simulink model "huamo"  (R2014a)
settings: Solver=ode3  SolverMode=SingleTasking  StartTime=0.0  StopTime=10.0  RelTol=1e-3
PreLoadFcn:
  | waijung.modelPreload; % Required for working with Waijung Blockset. Do not remove.
undefined symbols (not defined in the file): ARM, dfilt, DiscIntNeverNeededParam, fdesignblkfcn, gcbh, Link, LQFP64, MDK, ST, STM32F405RG
libraries: simulink x33, stm32f4_io_lib x3, stm32f4_device_config_lib x2, dsparch4 x2
(part 2 of 6)

== system huamo/IMU ==
  Bus Creator : BusCreator  Inputs=3
  Cal : Subsystem  TreatAsAtomicUnit=on
  Gain{1..4} (4 alike) : Gain  Gain=-1
  Mux : Mux  Inputs=3
  Mux1 : Mux  Inputs=3
  angle : S-Function  Priority=1  FunctionName=stm32f4_usart  Parameters=configuration,uartmodule,transfer,baudrate,inputtype,outputtype,confstr,binheaderarray,binterminatorarray,asciiheader,asciiterminator,bindatalength,packetmode,varname,sampletime,sampletimestr,blockid  EnableBusSupport=off  mask(stm32f4_usart){configuration=Rx, uartmodule=3, baudrate=115200, databits=8, parity=No, stopbit=1, remaptxpin=Not used, remaprxpin=Not used, flowcontrol=None, remapctspin=Not used, remaprtspin=Not used, advanceoptions=off, rxbuffersize=512, txbuffersize=512, transfer=Non-Blocking, packetmode=Binary, binheader='A5 5A 11 A4', binterminator='AA', porttype_double=0, porttype_single=0, porttype_int8=0, porttype_uint8=14, porttype_int16=0, porttype_uint16=0, porttype_int32=0, porttype_uint32=0, asciiformat='value=%d,%f', rx_asciiterminator=CRLF (0x0D 0x0A - "\r\n"), tx_asciiterminator=LF (0x0A - "\n"), storagename=<empty>, varname=, inputtype=[0], outputtype=[15 3  3 3 3 3 3 3 3 3 3 3 3 3 3 3], binheaderarray=[4 165   90   17  164    0    0    0    0    0    0    0    0    0    0    0    0    0    0    0    0    0    0    0    0], binterminatorarray=[1 170], bindatalength=14, asciiheader='value=%d,%f\r\n', asciiterminator=[2 13 10], sampletime=-1, sampletimestr=0.005, blockid=IMUangle, confstr=[ "dummy", "0", "*", "*", "0", "*", "*", "0", "*", "*", "0", "*", "*", "1", "4", "3", "1", "4", "1", "512", "512", "1", "3", "115200", "8", "No", "1", "None", "USART3"], lastmodule=1}
      mask prompts: uartmodule "UART Module"; baudrate "Baud rate (bps)"; databits "Data bits"; stopbit "Stop bit"; remaptxpin "Tx Pin"; remaprxpin "Rx Pin"; flowcontrol "Hardware flow control"; remapctspin "HW Flow control, CTS Pin"; remaprtspin "HW Flow control, RTS Pin"; advanceoptions "Advance options"; rxbuffersize "Rx buffer size (bytes)"; txbuffersize "Tx buffer size (bytes)"; packetmode "Packet mode"; binheader "Binary header (example: '7E 7E')"; binterminator "Binary terminator (example: '03 03')"; porttype_double "Number of data port, type DOUBLE"; porttype_single "Number of data port, type SINGLE"; porttype_int8 "Number of data port, type INT8"; porttype_uint8 "Number of data port, type UINT8"; porttype_int16 "Number of data port, type INT16"; porttype_uint16 "Number of data port, type UINT16"; porttype_int32 "Number of data port, type INT32"; porttype_uint32 "Number of data port, type UINT32"; asciiformat "Ascii format"; rx_asciiterminator "End of packet"; tx_asciiterminator "End of packet"; storagename "Buffer"; varname "Var name"; inputtype "Input data type"; outputtype "Output data type"; binheaderarray "Binary header"; binterminatorarray "Binary terminator"; bindatalength "Binary data length"; asciiheader "Ascii header (printf format)"; asciiterminator "Ascii terminator"; sampletime "Sample time (sec)"; sampletimestr "Compiled sample time (sec) in string"; confstr "Configuration string"; lastmodule "Last module selected"
      mask help:
      | Data type for Ascii format
      | %u, %i, %d, %o, %x: uint32
      | %e, %g, %f: single
      | %c: int8
      mask init:
      | stm32f4_usart_callback('init');
      mask Help: web(fullfile(waijungdocroot,'stm32f4_usart_rx.htm'), '-browser')
      mask TypeOptions configuration: Setup | Tx | Rx
      mask Callback configuration: stm32f4_usart_callback('configuration');
      mask TypeOptions uartmodule: 1 | 2 | 3 | 4 | 5 | 6
      mask Callback uartmodule: stm32f4_usart_callback('uartmodule');
      mask Callback baudrate: stm32f4_usart_callback('baudrate');
      mask TypeOptions databits: 8
      mask TypeOptions parity: No | Odd | Even
      mask TypeOptions stopbit: 0.5 | 1 | 1.5 | 2
      mask TypeOptions remaptxpin: Not used | A9 | B6
      mask TypeOptions remaprxpin: Not used | A10 | B7
      mask TypeOptions flowcontrol: None | RTS | CTS | RTS/CTS
      mask Callback flowcontrol: stm32f4_usart_callback('flowcontrol');
      mask TypeOptions remapctspin: Not used | A11
      mask TypeOptions remaprtspin: Not used | A12
      mask Callback advanceoptions: stm32f4_usart_callback('advanceoptions');
      mask TypeOptions rxbuffersize: 16 | 32 | 64 | 128 | 256 | 512 | 1024 | 2048
      mask TypeOptions txbuffersize: 16 | 32 | 64 | 128 | 256 | 512 | 1024 | 2048
      mask TypeOptions transfer: Blocking | Non-Blocking
      mask Callback transfer: stm32f4_usart_callback('transfer');
      mask TypeOptions packetmode: Ascii | Binary | String Buffer
      mask Callback packetmode: stm32f4_usart_callback('packetmode');
      mask Callback binheader: stm32f4_usart_callback('binheader');
      mask Callback binterminator: stm32f4_usart_callback('binterminator');
      mask Callback porttype_double: stm32f4_usart_callback('porttype');
      mask Callback porttype_single: stm32f4_usart_callback('porttype');
      mask Callback porttype_int8: stm32f4_usart_callback('porttype');
      mask Callback porttype_uint8: stm32f4_usart_callback('porttype');
      mask Callback porttype_int16: stm32f4_usart_callback('porttype');
      mask Callback porttype_uint16: stm32f4_usart_callback('porttype');
      mask Callback porttype_int32: stm32f4_usart_callback('porttype');
      mask Callback porttype_uint32: stm32f4_usart_callback('porttype');
      mask Callback asciiformat: stm32f4_usart_callback('asciiformat');
      mask TypeOptions rx_asciiterminator: CR (0x0D - "\r") | LF (0x0A - "\n") | CRLF (0x0D 0x0A - "\r\n")
      mask Callback rx_asciiterminator: stm32f4_usart_callback('rx_asciiterminator');
      mask TypeOptions tx_asciiterminator: CR (0x0D - "\r") | LF (0x0A - "\n") | CRLF (0x0D 0x0A - "\r\n") | None
      mask Callback tx_asciiterminator: stm32f4_usart_callback('tx_asciiterminator');
      mask TypeOptions storagename: <empty>
      mask Callback storagename: stm32f4_usart_callback('storagename');
      mask Callback varname: stm32f4_usart_callback('varname');
      mask Callback sampletime: stm32f4_usart_callback('sampletime');
      mask Callback sampletimestr: stm32f4_usart_callback('sampletimestr');
      mask Callback blockid: stm32f4_usart_callback('blockid');
      mask Display: text(0.05, 0.5, 'Module: USART3_Rx\nPacket: Binary\nTransfer: Non-Blocking\nTs (sec): 0.005','ver','middle','hor','left'); port_label('output', 1,'READY'); port_label('output', 2,'uint8'); port_label('output', 3,'uint8'); port_label('output', 4,'uint8'); port_label('output', 5,'uint8'); port_label('output', 6,'uint8'); port_label('output', 7,'uint8'); port_label('output', 8,'uint8'); port_label('output', 9,'uint8'); port_label('output', 10,'uint8'); port_label('output', 11,'uint8'); port_label('output', 12,'uint8'); port_label('output', 13,'uint8'); port_label('output', 14,'uint8'); port_label('output', 15,'uint8');
  ANGLE ENABLE : Outport
  IMU BUS : Outport  Port=2
  IMU : Outport  Port=3
  wires:
  angle/1 -> ANGLE ENABLE/1, Cal/Enable
  [alt] -> Bus Creator/3  "alt"
  [Angle_rate] -> Bus Creator/2  "Angle_rate"
  Mux/1 -> [Angle]  "angle"
  [Angle] -> Bus Creator/1  "Angle"
  Cal/2(pitch) -> Gain1/1
  Bus Creator/1 -> IMU BUS/1
  Gain2/1 -> Mux/3
  angle/2 -> Cal/1(yaw_H)
  angle/3 -> Cal/2(yaw_L)
  angle/4 -> Cal/3(pitch_H)
  angle/5 -> Cal/4(pitch_L)
  angle/6 -> Cal/5(roll_H)
  angle/7 -> Cal/6(roll_L)
  angle/8 -> Cal/7(p_H)
  angle/9 -> Cal/8(p_L)
  angle/10 -> Cal/9(q_H)
  angle/11 -> Cal/10(q_L)
  angle/12 -> Cal/11(r_H)
  angle/13 -> Cal/12(r_L)
  angle/14 -> Cal/13(alt_H)
  angle/15 -> Cal/14(alt_L)
  Gain1/1 -> Mux/2
  Mux1/1 -> [Angle_rate]  "angle"
  Cal/6(r) -> Gain4/1
  Cal/5(q) -> Gain3/1
  Cal/4(p) -> Mux1/1
  Gain4/1 -> Mux1/3
  Gain3/1 -> Mux1/2
  Cal/3(roll) -> Mux/1
  Cal/1(yaw) -> Gain2/1
  Cal/7(alt) -> [alt]
  Cal/8(out) -> IMU/1

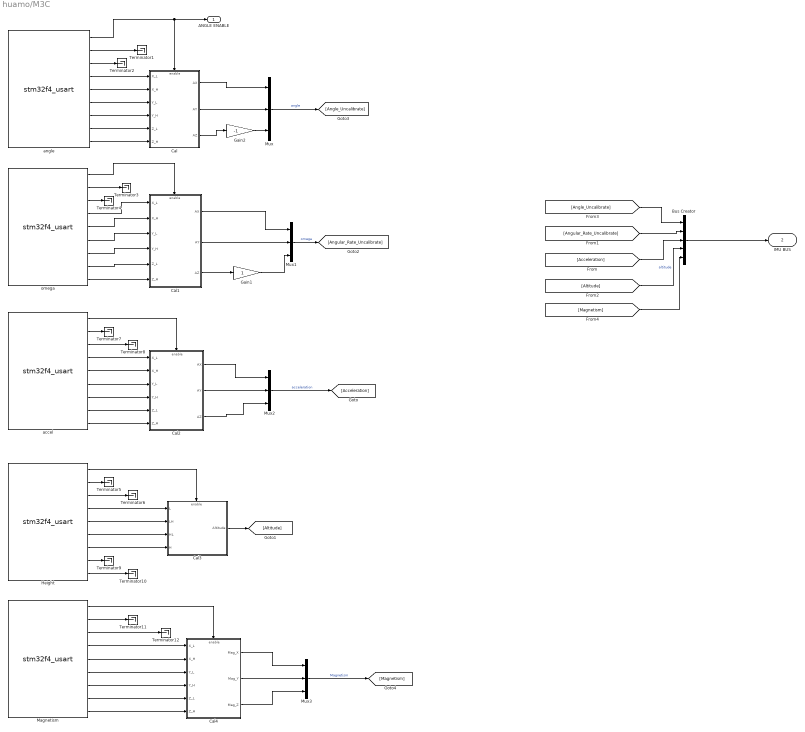
== system huamo/M3C ==
  Bus Creator : BusCreator  Inputs=5
  Cal : Subsystem  TreatAsAtomicUnit=on
  Cal1 : Subsystem  TreatAsAtomicUnit=on
  Cal2 : Subsystem  TreatAsAtomicUnit=on
  Cal3 : Subsystem  TreatAsAtomicUnit=on
  Cal4 : Subsystem  TreatAsAtomicUnit=on
  Gain1 : Gain
  Gain2 : Gain  Gain=-1
  Height : S-Function  Priority=1  FunctionName=stm32f4_usart  Parameters=configuration,uartmodule,transfer,baudrate,inputtype,outputtype,confstr,binheaderarray,binterminatorarray,asciiheader,asciiterminator,bindatalength,packetmode,varname,sampletime,sampletimestr,blockid  EnableBusSupport=off  mask(stm32f4_usart){configuration=Rx, uartmodule=3, baudrate=115200, databits=8, parity=No, stopbit=1, remaptxpin=Not used, remaprxpin=Not used, flowcontrol=None, remapctspin=Not used, remaprtspin=Not used, advanceoptions=off, rxbuffersize=512, txbuffersize=512, transfer=Non-Blocking, packetmode=Binary, binheader='A7 7A 75', binterminator='', porttype_double=0, porttype_single=0, porttype_int8=0, porttype_uint8=8, porttype_int16=0, porttype_uint16=0, porttype_int32=0, porttype_uint32=0, asciiformat='value=%d,%f', rx_asciiterminator=CRLF (0x0D 0x0A - "\r\n"), tx_asciiterminator=LF (0x0A - "\n"), storagename=<empty>, varname=, inputtype=[0], outputtype=[9 3  3 3 3 3 3 3 3 3], binheaderarray=[3 167  122  117    0    0    0], binterminatorarray=[0 ], bindatalength=8, asciiheader='value=%d,%f\r\n', asciiterminator=[2 13 10], sampletime=-1, sampletimestr=0.005, blockid=M3CHeight, confstr=[ "dummy", "0", "*", "*", "0", "*", "*", "0", "*", "*", "0", "*", "*", "1", "4", "3", "1", "4", "1", "512", "512", "1", "3", "115200", "8", "No", "1", "None", "USART3"], lastmodule=1}
      mask prompts: uartmodule "UART Module"; baudrate "Baud rate (bps)"; databits "Data bits"; stopbit "Stop bit"; remaptxpin "Tx Pin"; remaprxpin "Rx Pin"; flowcontrol "Hardware flow control"; remapctspin "HW Flow control, CTS Pin"; remaprtspin "HW Flow control, RTS Pin"; advanceoptions "Advance options"; rxbuffersize "Rx buffer size (bytes)"; txbuffersize "Tx buffer size (bytes)"; packetmode "Packet mode"; binheader "Binary header (example: '7E 7E')"; binterminator "Binary terminator (example: '03 03')"; porttype_double "Number of data port, type DOUBLE"; porttype_single "Number of data port, type SINGLE"; porttype_int8 "Number of data port, type INT8"; porttype_uint8 "Number of data port, type UINT8"; porttype_int16 "Number of data port, type INT16"; porttype_uint16 "Number of data port, type UINT16"; porttype_int32 "Number of data port, type INT32"; porttype_uint32 "Number of data port, type UINT32"; asciiformat "Ascii format"; rx_asciiterminator "End of packet"; tx_asciiterminator "End of packet"; storagename "Buffer"; varname "Var name"; inputtype "Input data type"; outputtype "Output data type"; binheaderarray "Binary header"; binterminatorarray "Binary terminator"; bindatalength "Binary data length"; asciiheader "Ascii header (printf format)"; asciiterminator "Ascii terminator"; sampletime "Sample time (sec)"; sampletimestr "Compiled sample time (sec) in string"; confstr "Configuration string"; lastmodule "Last module selected"
      mask help:
      | Data type for Ascii format
      | %u, %i, %d, %o, %x: uint32
      | %e, %g, %f: single
      | %c: int8
      mask init:
      | stm32f4_usart_callback('init');
      mask Help: web(fullfile(waijungdocroot,'stm32f4_usart_rx.htm'), '-browser')
      mask TypeOptions configuration: Setup | Tx | Rx
      mask Callback configuration: stm32f4_usart_callback('configuration');
      mask TypeOptions uartmodule: 1 | 2 | 3 | 4 | 5 | 6
      mask Callback uartmodule: stm32f4_usart_callback('uartmodule');
      mask Callback baudrate: stm32f4_usart_callback('baudrate');
      mask TypeOptions databits: 8
      mask TypeOptions parity: No | Odd | Even
      mask TypeOptions stopbit: 0.5 | 1 | 1.5 | 2
      mask TypeOptions remaptxpin: Not used | A9 | B6
      mask TypeOptions remaprxpin: Not used | A10 | B7
      mask TypeOptions flowcontrol: None | RTS | CTS | RTS/CTS
      mask Callback flowcontrol: stm32f4_usart_callback('flowcontrol');
      mask TypeOptions remapctspin: Not used | A11
      mask TypeOptions remaprtspin: Not used | A12
      mask Callback advanceoptions: stm32f4_usart_callback('advanceoptions');
      mask TypeOptions rxbuffersize: 16 | 32 | 64 | 128 | 256 | 512 | 1024 | 2048
      mask TypeOptions txbuffersize: 16 | 32 | 64 | 128 | 256 | 512 | 1024 | 2048
      mask TypeOptions transfer: Blocking | Non-Blocking
      mask Callback transfer: stm32f4_usart_callback('transfer');
      mask TypeOptions packetmode: Ascii | Binary | String Buffer
      mask Callback packetmode: stm32f4_usart_callback('packetmode');
      mask Callback binheader: stm32f4_usart_callback('binheader');
      mask Callback binterminator: stm32f4_usart_callback('binterminator');
      mask Callback porttype_double: stm32f4_usart_callback('porttype');
      mask Callback porttype_single: stm32f4_usart_callback('porttype');
      mask Callback porttype_int8: stm32f4_usart_callback('porttype');
      mask Callback porttype_uint8: stm32f4_usart_callback('porttype');
      mask Callback porttype_int16: stm32f4_usart_callback('porttype');
      mask Callback porttype_uint16: stm32f4_usart_callback('porttype');
      mask Callback porttype_int32: stm32f4_usart_callback('porttype');
      mask Callback porttype_uint32: stm32f4_usart_callback('porttype');
      mask Callback asciiformat: stm32f4_usart_callback('asciiformat');
      mask TypeOptions rx_asciiterminator: CR (0x0D - "\r") | LF (0x0A - "\n") | CRLF (0x0D 0x0A - "\r\n")
      mask Callback rx_asciiterminator: stm32f4_usart_callback('rx_asciiterminator');
      mask TypeOptions tx_asciiterminator: CR (0x0D - "\r") | LF (0x0A - "\n") | CRLF (0x0D 0x0A - "\r\n") | None
      mask Callback tx_asciiterminator: stm32f4_usart_callback('tx_asciiterminator');
      mask TypeOptions storagename: <empty>
      mask Callback storagename: stm32f4_usart_callback('storagename');
      mask Callback varname: stm32f4_usart_callback('varname');
      mask Callback sampletime: stm32f4_usart_callback('sampletime');
      mask Callback sampletimestr: stm32f4_usart_callback('sampletimestr');
      mask Callback blockid: stm32f4_usart_callback('blockid');
      mask Display: text(0.05, 0.5, 'Module: USART3_Rx\nPacket: Binary\nTransfer: Non-Blocking\nTs (sec): 0.005','ver','middle','hor','left'); port_label('output', 1,'READY'); port_label('output', 2,'uint8'); port_label('output', 3,'uint8'); port_label('output', 4,'uint8'); port_label('output', 5,'uint8'); port_label('output', 6,'uint8'); port_label('output', 7,'uint8'); port_label('output', 8,'uint8'); port_label('output', 9,'uint8');
  Magnetism : S-Function  Priority=1  FunctionName=stm32f4_usart  Parameters=configuration,uartmodule,transfer,baudrate,inputtype,outputtype,confstr,binheaderarray,binterminatorarray,asciiheader,asciiterminator,bindatalength,packetmode,varname,sampletime,sampletimestr,blockid  EnableBusSupport=off  mask(stm32f4_usart){configuration=Rx, uartmodule=3, baudrate=115200, databits=8, parity=No, stopbit=1, remaptxpin=Not used, remaprxpin=Not used, flowcontrol=None, remapctspin=Not used, remaprtspin=Not used, advanceoptions=off, rxbuffersize=512, txbuffersize=512, transfer=Non-Blocking, packetmode=Binary, binheader='A7 7A 73', binterminator='', porttype_double=0, porttype_single=0, porttype_int8=0, porttype_uint8=8, porttype_int16=0, porttype_uint16=0, porttype_int32=0, porttype_uint32=0, asciiformat='value=%d,%f', rx_asciiterminator=CRLF (0x0D 0x0A - "\r\n"), tx_asciiterminator=LF (0x0A - "\n"), storagename=<empty>, varname=, inputtype=[0], outputtype=[9 3  3 3 3 3 3 3 3 3], binheaderarray=[3 167  122  115    0    0    0], binterminatorarray=[0 ], bindatalength=8, asciiheader='value=%d,%f\r\n', asciiterminator=[2 13 10], sampletime=-1, sampletimestr=0.005, blockid=M3CMagnetism, confstr=[ "dummy", "0", "*", "*", "0", "*", "*", "0", "*", "*", "0", "*", "*", "1", "4", "3", "1", "4", "1", "512", "512", "1", "3", "115200", "8", "No", "1", "None", "USART3"], lastmodule=1}
      mask prompts: uartmodule "UART Module"; baudrate "Baud rate (bps)"; databits "Data bits"; stopbit "Stop bit"; remaptxpin "Tx Pin"; remaprxpin "Rx Pin"; flowcontrol "Hardware flow control"; remapctspin "HW Flow control, CTS Pin"; remaprtspin "HW Flow control, RTS Pin"; advanceoptions "Advance options"; rxbuffersize "Rx buffer size (bytes)"; txbuffersize "Tx buffer size (bytes)"; packetmode "Packet mode"; binheader "Binary header (example: '7E 7E')"; binterminator "Binary terminator (example: '03 03')"; porttype_double "Number of data port, type DOUBLE"; porttype_single "Number of data port, type SINGLE"; porttype_int8 "Number of data port, type INT8"; porttype_uint8 "Number of data port, type UINT8"; porttype_int16 "Number of data port, type INT16"; porttype_uint16 "Number of data port, type UINT16"; porttype_int32 "Number of data port, type INT32"; porttype_uint32 "Number of data port, type UINT32"; asciiformat "Ascii format"; rx_asciiterminator "End of packet"; tx_asciiterminator "End of packet"; storagename "Buffer"; varname "Var name"; inputtype "Input data type"; outputtype "Output data type"; binheaderarray "Binary header"; binterminatorarray "Binary terminator"; bindatalength "Binary data length"; asciiheader "Ascii header (printf format)"; asciiterminator "Ascii terminator"; sampletime "Sample time (sec)"; sampletimestr "Compiled sample time (sec) in string"; confstr "Configuration string"; lastmodule "Last module selected"
      mask help:
      | Data type for Ascii format
      | %u, %i, %d, %o, %x: uint32
      | %e, %g, %f: single
      | %c: int8
      mask init:
      | stm32f4_usart_callback('init');
      mask Help: web(fullfile(waijungdocroot,'stm32f4_usart_rx.htm'), '-browser')
      mask TypeOptions configuration: Setup | Tx | Rx
      mask Callback configuration: stm32f4_usart_callback('configuration');
      mask TypeOptions uartmodule: 1 | 2 | 3 | 4 | 5 | 6
      mask Callback uartmodule: stm32f4_usart_callback('uartmodule');
      mask Callback baudrate: stm32f4_usart_callback('baudrate');
      mask TypeOptions databits: 8
      mask TypeOptions parity: No | Odd | Even
      mask TypeOptions stopbit: 0.5 | 1 | 1.5 | 2
      mask TypeOptions remaptxpin: Not used | A9 | B6
      mask TypeOptions remaprxpin: Not used | A10 | B7
      mask TypeOptions flowcontrol: None | RTS | CTS | RTS/CTS
      mask Callback flowcontrol: stm32f4_usart_callback('flowcontrol');
      mask TypeOptions remapctspin: Not used | A11
      mask TypeOptions remaprtspin: Not used | A12
      mask Callback advanceoptions: stm32f4_usart_callback('advanceoptions');
      mask TypeOptions rxbuffersize: 16 | 32 | 64 | 128 | 256 | 512 | 1024 | 2048
      mask TypeOptions txbuffersize: 16 | 32 | 64 | 128 | 256 | 512 | 1024 | 2048
      mask TypeOptions transfer: Blocking | Non-Blocking
      mask Callback transfer: stm32f4_usart_callback('transfer');
      mask TypeOptions packetmode: Ascii | Binary | String Buffer
      mask Callback packetmode: stm32f4_usart_callback('packetmode');
      mask Callback binheader: stm32f4_usart_callback('binheader');
      mask Callback binterminator: stm32f4_usart_callback('binterminator');
      mask Callback porttype_double: stm32f4_usart_callback('porttype');
      mask Callback porttype_single: stm32f4_usart_callback('porttype');
      mask Callback porttype_int8: stm32f4_usart_callback('porttype');
      mask Callback porttype_uint8: stm32f4_usart_callback('porttype');
      mask Callback porttype_int16: stm32f4_usart_callback('porttype');
      mask Callback porttype_uint16: stm32f4_usart_callback('porttype');
      mask Callback porttype_int32: stm32f4_usart_callback('porttype');
      mask Callback porttype_uint32: stm32f4_usart_callback('porttype');
      mask Callback asciiformat: stm32f4_usart_callback('asciiformat');
      mask TypeOptions rx_asciiterminator: CR (0x0D - "\r") | LF (0x0A - "\n") | CRLF (0x0D 0x0A - "\r\n")
      mask Callback rx_asciiterminator: stm32f4_usart_callback('rx_asciiterminator');
      mask TypeOptions tx_asciiterminator: CR (0x0D - "\r") | LF (0x0A - "\n") | CRLF (0x0D 0x0A - "\r\n") | None
      mask Callback tx_asciiterminator: stm32f4_usart_callback('tx_asciiterminator');
      mask TypeOptions storagename: <empty>
      mask Callback storagename: stm32f4_usart_callback('storagename');
      mask Callback varname: stm32f4_usart_callback('varname');
      mask Callback sampletime: stm32f4_usart_callback('sampletime');
      mask Callback sampletimestr: stm32f4_usart_callback('sampletimestr');
      mask Callback blockid: stm32f4_usart_callback('blockid');
      mask Display: text(0.05, 0.5, 'Module: USART3_Rx\nPacket: Binary\nTransfer: Non-Blocking\nTs (sec): 0.005','ver','middle','hor','left'); port_label('output', 1,'READY'); port_label('output', 2,'uint8'); port_label('output', 3,'uint8'); port_label('output', 4,'uint8'); port_label('output', 5,'uint8'); port_label('output', 6,'uint8'); port_label('output', 7,'uint8'); port_label('output', 8,'uint8'); port_label('output', 9,'uint8');
  Mux{,1..3} (4 alike) : Mux  Inputs=3
  Terminator{1..12} (12 alike) : Terminator
  accel : S-Function  Priority=1  FunctionName=stm32f4_usart  Parameters=configuration,uartmodule,transfer,baudrate,inputtype,outputtype,confstr,binheaderarray,binterminatorarray,asciiheader,asciiterminator,bindatalength,packetmode,varname,sampletime,sampletimestr,blockid  EnableBusSupport=off  mask(stm32f4_usart){configuration=Rx, uartmodule=3, baudrate=115200, databits=8, parity=No, stopbit=1, remaptxpin=Not used, remaprxpin=Not used, flowcontrol=None, remapctspin=Not used, remaprtspin=Not used, advanceoptions=off, rxbuffersize=512, txbuffersize=512, transfer=Non-Blocking, packetmode=Binary, binheader='A7 7A 71', binterminator='', porttype_double=0, porttype_single=0, porttype_int8=0, porttype_uint8=8, porttype_int16=0, porttype_uint16=0, porttype_int32=0, porttype_uint32=0, asciiformat='value=%d,%f', rx_asciiterminator=CRLF (0x0D 0x0A - "\r\n"), tx_asciiterminator=LF (0x0A - "\n"), storagename=<empty>, varname=, inputtype=[0], outputtype=[9 3  3 3 3 3 3 3 3 3], binheaderarray=[3 167  122  113    0    0    0], binterminatorarray=[0 ], bindatalength=8, asciiheader='value=%d,%f\r\n', asciiterminator=[2 13 10], sampletime=-1, sampletimestr=0.005, blockid=M3Caccel, confstr=[ "dummy", "0", "*", "*", "0", "*", "*", "0", "*", "*", "0", "*", "*", "1", "4", "3", "1", "4", "1", "512", "512", "1", "3", "115200", "8", "No", "1", "None", "USART3"], lastmodule=1}
      mask prompts: uartmodule "UART Module"; baudrate "Baud rate (bps)"; databits "Data bits"; stopbit "Stop bit"; remaptxpin "Tx Pin"; remaprxpin "Rx Pin"; flowcontrol "Hardware flow control"; remapctspin "HW Flow control, CTS Pin"; remaprtspin "HW Flow control, RTS Pin"; advanceoptions "Advance options"; rxbuffersize "Rx buffer size (bytes)"; txbuffersize "Tx buffer size (bytes)"; packetmode "Packet mode"; binheader "Binary header (example: '7E 7E')"; binterminator "Binary terminator (example: '03 03')"; porttype_double "Number of data port, type DOUBLE"; porttype_single "Number of data port, type SINGLE"; porttype_int8 "Number of data port, type INT8"; porttype_uint8 "Number of data port, type UINT8"; porttype_int16 "Number of data port, type INT16"; porttype_uint16 "Number of data port, type UINT16"; porttype_int32 "Number of data port, type INT32"; porttype_uint32 "Number of data port, type UINT32"; asciiformat "Ascii format"; rx_asciiterminator "End of packet"; tx_asciiterminator "End of packet"; storagename "Buffer"; varname "Var name"; inputtype "Input data type"; outputtype "Output data type"; binheaderarray "Binary header"; binterminatorarray "Binary terminator"; bindatalength "Binary data length"; asciiheader "Ascii header (printf format)"; asciiterminator "Ascii terminator"; sampletime "Sample time (sec)"; sampletimestr "Compiled sample time (sec) in string"; confstr "Configuration string"; lastmodule "Last module selected"
      mask help:
      | Data type for Ascii format
      | %u, %i, %d, %o, %x: uint32
      | %e, %g, %f: single
      | %c: int8
      mask init:
      | stm32f4_usart_callback('init');
      mask Help: web(fullfile(waijungdocroot,'stm32f4_usart_rx.htm'), '-browser')
      mask TypeOptions configuration: Setup | Tx | Rx
      mask Callback configuration: stm32f4_usart_callback('configuration');
      mask TypeOptions uartmodule: 1 | 2 | 3 | 4 | 5 | 6
      mask Callback uartmodule: stm32f4_usart_callback('uartmodule');
      mask Callback baudrate: stm32f4_usart_callback('baudrate');
      mask TypeOptions databits: 8
      mask TypeOptions parity: No | Odd | Even
      mask TypeOptions stopbit: 0.5 | 1 | 1.5 | 2
      mask TypeOptions remaptxpin: Not used | A9 | B6
      mask TypeOptions remaprxpin: Not used | A10 | B7
      mask TypeOptions flowcontrol: None | RTS | CTS | RTS/CTS
      mask Callback flowcontrol: stm32f4_usart_callback('flowcontrol');
      mask TypeOptions remapctspin: Not used | A11
      mask TypeOptions remaprtspin: Not used | A12
      mask Callback advanceoptions: stm32f4_usart_callback('advanceoptions');
      mask TypeOptions rxbuffersize: 16 | 32 | 64 | 128 | 256 | 512 | 1024 | 2048
      mask TypeOptions txbuffersize: 16 | 32 | 64 | 128 | 256 | 512 | 1024 | 2048
      mask TypeOptions transfer: Blocking | Non-Blocking
      mask Callback transfer: stm32f4_usart_callback('transfer');
      mask TypeOptions packetmode: Ascii | Binary | String Buffer
      mask Callback packetmode: stm32f4_usart_callback('packetmode');
      mask Callback binheader: stm32f4_usart_callback('binheader');
      mask Callback binterminator: stm32f4_usart_callback('binterminator');
      mask Callback porttype_double: stm32f4_usart_callback('porttype');
      mask Callback porttype_single: stm32f4_usart_callback('porttype');
      mask Callback porttype_int8: stm32f4_usart_callback('porttype');
      mask Callback porttype_uint8: stm32f4_usart_callback('porttype');
      mask Callback porttype_int16: stm32f4_usart_callback('porttype');
      mask Callback porttype_uint16: stm32f4_usart_callback('porttype');
      mask Callback porttype_int32: stm32f4_usart_callback('porttype');
      mask Callback porttype_uint32: stm32f4_usart_callback('porttype');
      mask Callback asciiformat: stm32f4_usart_callback('asciiformat');
      mask TypeOptions rx_asciiterminator: CR (0x0D - "\r") | LF (0x0A - "\n") | CRLF (0x0D 0x0A - "\r\n")
      mask Callback rx_asciiterminator: stm32f4_usart_callback('rx_asciiterminator');
      mask TypeOptions tx_asciiterminator: CR (0x0D - "\r") | LF (0x0A - "\n") | CRLF (0x0D 0x0A - "\r\n") | None
      mask Callback tx_asciiterminator: stm32f4_usart_callback('tx_asciiterminator');
      mask TypeOptions storagename: <empty>
      mask Callback storagename: stm32f4_usart_callback('storagename');
      mask Callback varname: stm32f4_usart_callback('varname');
      mask Callback sampletime: stm32f4_usart_callback('sampletime');
      mask Callback sampletimestr: stm32f4_usart_callback('sampletimestr');
      mask Callback blockid: stm32f4_usart_callback('blockid');
      mask Display: text(0.05, 0.5, 'Module: USART3_Rx\nPacket: Binary\nTransfer: Non-Blocking\nTs (sec): 0.005','ver','middle','hor','left'); port_label('output', 1,'READY'); port_label('output', 2,'uint8'); port_label('output', 3,'uint8'); port_label('output', 4,'uint8'); port_label('output', 5,'uint8'); port_label('output', 6,'uint8'); port_label('output', 7,'uint8'); port_label('output', 8,'uint8'); port_label('output', 9,'uint8');
  angle : S-Function  Priority=1  FunctionName=stm32f4_usart  Parameters=configuration,uartmodule,transfer,baudrate,inputtype,outputtype,confstr,binheaderarray,binterminatorarray,asciiheader,asciiterminator,bindatalength,packetmode,varname,sampletime,sampletimestr,blockid  EnableBusSupport=off  mask(stm32f4_usart){configuration=Rx, uartmodule=3, baudrate=115200, databits=8, parity=No, stopbit=1, remaptxpin=Not used, remaprxpin=Not used, flowcontrol=None, remapctspin=Not used, remaprtspin=Not used, advanceoptions=off, rxbuffersize=512, txbuffersize=512, transfer=Non-Blocking, packetmode=Binary, binheader='A7 7A 72', binterminator='', porttype_double=0, porttype_single=0, porttype_int8=0, porttype_uint8=8, porttype_int16=0, porttype_uint16=0, porttype_int32=0, porttype_uint32=0, asciiformat='value=%d,%f', rx_asciiterminator=CRLF (0x0D 0x0A - "\r\n"), tx_asciiterminator=LF (0x0A - "\n"), storagename=<empty>, varname=, inputtype=[0], outputtype=[9 3  3 3 3 3 3 3 3 3], binheaderarray=[3 167  122  114    0    0    0], binterminatorarray=[0 ], bindatalength=8, asciiheader='value=%d,%f\r\n', asciiterminator=[2 13 10], sampletime=-1, sampletimestr=0.005, blockid=M3Cangle, confstr=[ "dummy", "0", "*", "*", "0", "*", "*", "0", "*", "*", "0", "*", "*", "1", "4", "3", "1", "4", "1", "512", "512", "1", "3", "115200", "8", "No", "1", "None", "USART3"], lastmodule=1}
      mask prompts: uartmodule "UART Module"; baudrate "Baud rate (bps)"; databits "Data bits"; stopbit "Stop bit"; remaptxpin "Tx Pin"; remaprxpin "Rx Pin"; flowcontrol "Hardware flow control"; remapctspin "HW Flow control, CTS Pin"; remaprtspin "HW Flow control, RTS Pin"; advanceoptions "Advance options"; rxbuffersize "Rx buffer size (bytes)"; txbuffersize "Tx buffer size (bytes)"; packetmode "Packet mode"; binheader "Binary header (example: '7E 7E')"; binterminator "Binary terminator (example: '03 03')"; porttype_double "Number of data port, type DOUBLE"; porttype_single "Number of data port, type SINGLE"; porttype_int8 "Number of data port, type INT8"; porttype_uint8 "Number of data port, type UINT8"; porttype_int16 "Number of data port, type INT16"; porttype_uint16 "Number of data port, type UINT16"; porttype_int32 "Number of data port, type INT32"; porttype_uint32 "Number of data port, type UINT32"; asciiformat "Ascii format"; rx_asciiterminator "End of packet"; tx_asciiterminator "End of packet"; storagename "Buffer"; varname "Var name"; inputtype "Input data type"; outputtype "Output data type"; binheaderarray "Binary header"; binterminatorarray "Binary terminator"; bindatalength "Binary data length"; asciiheader "Ascii header (printf format)"; asciiterminator "Ascii terminator"; sampletime "Sample time (sec)"; sampletimestr "Compiled sample time (sec) in string"; confstr "Configuration string"; lastmodule "Last module selected"
      mask help:
      | Data type for Ascii format
      | %u, %i, %d, %o, %x: uint32
      | %e, %g, %f: single
      | %c: int8
      mask init:
      | stm32f4_usart_callback('init');
      mask Help: web(fullfile(waijungdocroot,'stm32f4_usart_rx.htm'), '-browser')
      mask TypeOptions configuration: Setup | Tx | Rx
      mask Callback configuration: stm32f4_usart_callback('configuration');
      mask TypeOptions uartmodule: 1 | 2 | 3 | 4 | 5 | 6
      mask Callback uartmodule: stm32f4_usart_callback('uartmodule');
      mask Callback baudrate: stm32f4_usart_callback('baudrate');
      mask TypeOptions databits: 8
      mask TypeOptions parity: No | Odd | Even
      mask TypeOptions stopbit: 0.5 | 1 | 1.5 | 2
      mask TypeOptions remaptxpin: Not used | A9 | B6
      mask TypeOptions remaprxpin: Not used | A10 | B7
      mask TypeOptions flowcontrol: None | RTS | CTS | RTS/CTS
      mask Callback flowcontrol: stm32f4_usart_callback('flowcontrol');
      mask TypeOptions remapctspin: Not used | A11
      mask TypeOptions remaprtspin: Not used | A12
      mask Callback advanceoptions: stm32f4_usart_callback('advanceoptions');
      mask TypeOptions rxbuffersize: 16 | 32 | 64 | 128 | 256 | 512 | 1024 | 2048
      mask TypeOptions txbuffersize: 16 | 32 | 64 | 128 | 256 | 512 | 1024 | 2048
      mask TypeOptions transfer: Blocking | Non-Blocking
      mask Callback transfer: stm32f4_usart_callback('transfer');
      mask TypeOptions packetmode: Ascii | Binary | String Buffer
      mask Callback packetmode: stm32f4_usart_callback('packetmode');
      mask Callback binheader: stm32f4_usart_callback('binheader');
      mask Callback binterminator: stm32f4_usart_callback('binterminator');
      mask Callback porttype_double: stm32f4_usart_callback('porttype');
      mask Callback porttype_single: stm32f4_usart_callback('porttype');
      mask Callback porttype_int8: stm32f4_usart_callback('porttype');
      mask Callback porttype_uint8: stm32f4_usart_callback('porttype');
      mask Callback porttype_int16: stm32f4_usart_callback('porttype');
      mask Callback porttype_uint16: stm32f4_usart_callback('porttype');
      mask Callback porttype_int32: stm32f4_usart_callback('porttype');
      mask Callback porttype_uint32: stm32f4_usart_callback('porttype');
      mask Callback asciiformat: stm32f4_usart_callback('asciiformat');
      mask TypeOptions rx_asciiterminator: CR (0x0D - "\r") | LF (0x0A - "\n") | CRLF (0x0D 0x0A - "\r\n")
      mask Callback rx_asciiterminator: stm32f4_usart_callback('rx_asciiterminator');
      mask TypeOptions tx_asciiterminator: CR (0x0D - "\r") | LF (0x0A - "\n") | CRLF (0x0D 0x0A - "\r\n") | None
      mask Callback tx_asciiterminator: stm32f4_usart_callback('tx_asciiterminator');
      mask TypeOptions storagename: <empty>
      mask Callback storagename: stm32f4_usart_callback('storagename');
      mask Callback varname: stm32f4_usart_callback('varname');
      mask Callback sampletime: stm32f4_usart_callback('sampletime');
      mask Callback sampletimestr: stm32f4_usart_callback('sampletimestr');
      mask Callback blockid: stm32f4_usart_callback('blockid');
      mask Display: text(0.05, 0.5, 'Module: USART3_Rx\nPacket: Binary\nTransfer: Non-Blocking\nTs (sec): 0.005','ver','middle','hor','left'); port_label('output', 1,'READY'); port_label('output', 2,'uint8'); port_label('output', 3,'uint8'); port_label('output', 4,'uint8'); port_label('output', 5,'uint8'); port_label('output', 6,'uint8'); port_label('output', 7,'uint8'); port_label('output', 8,'uint8'); port_label('output', 9,'uint8');
  omega : S-Function  Priority=1  FunctionName=stm32f4_usart  Parameters=configuration,uartmodule,transfer,baudrate,inputtype,outputtype,confstr,binheaderarray,binterminatorarray,asciiheader,asciiterminator,bindatalength,packetmode,varname,sampletime,sampletimestr,blockid  EnableBusSupport=off  mask(stm32f4_usart){configuration=Rx, uartmodule=3, baudrate=115200, databits=8, parity=No, stopbit=1, remaptxpin=Not used, remaprxpin=Not used, flowcontrol=None, remapctspin=Not used, remaprtspin=Not used, advanceoptions=off, rxbuffersize=512, txbuffersize=512, transfer=Non-Blocking, packetmode=Binary, binheader='A7 7A 70', binterminator='', porttype_double=0, porttype_single=0, porttype_int8=0, porttype_uint8=8, porttype_int16=0, porttype_uint16=0, porttype_int32=0, porttype_uint32=0, asciiformat='value=%d,%f', rx_asciiterminator=CRLF (0x0D 0x0A - "\r\n"), tx_asciiterminator=LF (0x0A - "\n"), storagename=<empty>, varname=, inputtype=[0], outputtype=[9 3  3 3 3 3 3 3 3 3], binheaderarray=[3 167  122  112    0    0    0], binterminatorarray=[0 ], bindatalength=8, asciiheader='value=%d,%f\r\n', asciiterminator=[2 13 10], sampletime=-1, sampletimestr=0.005, blockid=M3Comega, confstr=[ "dummy", "0", "*", "*", "0", "*", "*", "0", "*", "*", "0", "*", "*", "1", "4", "3", "1", "4", "1", "512", "512", "1", "3", "115200", "8", "No", "1", "None", "USART3"], lastmodule=1}
      mask prompts: uartmodule "UART Module"; baudrate "Baud rate (bps)"; databits "Data bits"; stopbit "Stop bit"; remaptxpin "Tx Pin"; remaprxpin "Rx Pin"; flowcontrol "Hardware flow control"; remapctspin "HW Flow control, CTS Pin"; remaprtspin "HW Flow control, RTS Pin"; advanceoptions "Advance options"; rxbuffersize "Rx buffer size (bytes)"; txbuffersize "Tx buffer size (bytes)"; packetmode "Packet mode"; binheader "Binary header (example: '7E 7E')"; binterminator "Binary terminator (example: '03 03')"; porttype_double "Number of data port, type DOUBLE"; porttype_single "Number of data port, type SINGLE"; porttype_int8 "Number of data port, type INT8"; porttype_uint8 "Number of data port, type UINT8"; porttype_int16 "Number of data port, type INT16"; porttype_uint16 "Number of data port, type UINT16"; porttype_int32 "Number of data port, type INT32"; porttype_uint32 "Number of data port, type UINT32"; asciiformat "Ascii format"; rx_asciiterminator "End of packet"; tx_asciiterminator "End of packet"; storagename "Buffer"; varname "Var name"; inputtype "Input data type"; outputtype "Output data type"; binheaderarray "Binary header"; binterminatorarray "Binary terminator"; bindatalength "Binary data length"; asciiheader "Ascii header (printf format)"; asciiterminator "Ascii terminator"; sampletime "Sample time (sec)"; sampletimestr "Compiled sample time (sec) in string"; confstr "Configuration string"; lastmodule "Last module selected"
      mask help:
      | Data type for Ascii format
      | %u, %i, %d, %o, %x: uint32
      | %e, %g, %f: single
      | %c: int8
      mask init:
      | stm32f4_usart_callback('init');
      mask Help: web(fullfile(waijungdocroot,'stm32f4_usart_rx.htm'), '-browser')
      mask TypeOptions configuration: Setup | Tx | Rx
      mask Callback configuration: stm32f4_usart_callback('configuration');
      mask TypeOptions uartmodule: 1 | 2 | 3 | 4 | 5 | 6
      mask Callback uartmodule: stm32f4_usart_callback('uartmodule');
      mask Callback baudrate: stm32f4_usart_callback('baudrate');
      mask TypeOptions databits: 8
      mask TypeOptions parity: No | Odd | Even
      mask TypeOptions stopbit: 0.5 | 1 | 1.5 | 2
      mask TypeOptions remaptxpin: Not used | A9 | B6
      mask TypeOptions remaprxpin: Not used | A10 | B7
      mask TypeOptions flowcontrol: None | RTS | CTS | RTS/CTS
      mask Callback flowcontrol: stm32f4_usart_callback('flowcontrol');
      mask TypeOptions remapctspin: Not used | A11
      mask TypeOptions remaprtspin: Not used | A12
      mask Callback advanceoptions: stm32f4_usart_callback('advanceoptions');
      mask TypeOptions rxbuffersize: 16 | 32 | 64 | 128 | 256 | 512 | 1024 | 2048
      mask TypeOptions txbuffersize: 16 | 32 | 64 | 128 | 256 | 512 | 1024 | 2048
      mask TypeOptions transfer: Blocking | Non-Blocking
      mask Callback transfer: stm32f4_usart_callback('transfer');
      mask TypeOptions packetmode: Ascii | Binary | String Buffer
      mask Callback packetmode: stm32f4_usart_callback('packetmode');
      mask Callback binheader: stm32f4_usart_callback('binheader');
      mask Callback binterminator: stm32f4_usart_callback('binterminator');
      mask Callback porttype_double: stm32f4_usart_callback('porttype');
      mask Callback porttype_single: stm32f4_usart_callback('porttype');
      mask Callback porttype_int8: stm32f4_usart_callback('porttype');
      mask Callback porttype_uint8: stm32f4_usart_callback('porttype');
      mask Callback porttype_int16: stm32f4_usart_callback('porttype');
      mask Callback porttype_uint16: stm32f4_usart_callback('porttype');
      mask Callback porttype_int32: stm32f4_usart_callback('porttype');
      mask Callback porttype_uint32: stm32f4_usart_callback('porttype');
      mask Callback asciiformat: stm32f4_usart_callback('asciiformat');
      mask TypeOptions rx_asciiterminator: CR (0x0D - "\r") | LF (0x0A - "\n") | CRLF (0x0D 0x0A - "\r\n")
      mask Callback rx_asciiterminator: stm32f4_usart_callback('rx_asciiterminator');
      mask TypeOptions tx_asciiterminator: CR (0x0D - "\r") | LF (0x0A - "\n") | CRLF (0x0D 0x0A - "\r\n") | None
      mask Callback tx_asciiterminator: stm32f4_usart_callback('tx_asciiterminator');
      mask TypeOptions storagename: <empty>
      mask Callback storagename: stm32f4_usart_callback('storagename');
      mask Callback varname: stm32f4_usart_callback('varname');
      mask Callback sampletime: stm32f4_usart_callback('sampletime');
      mask Callback sampletimestr: stm32f4_usart_callback('sampletimestr');
      mask Callback blockid: stm32f4_usart_callback('blockid');
      mask Display: text(0.05, 0.5, 'Module: USART3_Rx\nPacket: Binary\nTransfer: Non-Blocking\nTs (sec): 0.005','ver','middle','hor','left'); port_label('output', 1,'READY'); port_label('output', 2,'uint8'); port_label('output', 3,'uint8'); port_label('output', 4,'uint8'); port_label('output', 5,'uint8'); port_label('output', 6,'uint8'); port_label('output', 7,'uint8'); port_label('output', 8,'uint8'); port_label('output', 9,'uint8');
  ANGLE ENABLE : Outport
  IMU BUS : Outport  Port=2
  wires:
  angle/1 -> ANGLE ENABLE/1, Cal/Enable
  omega/1 -> Cal1/Enable
  Cal1/3(AZ) -> Gain1/1
  angle/3 -> Terminator2/1
  accel/1 -> Cal2/Enable
  Cal2/1(AX) -> Mux2/1
  Cal2/2(AY) -> Mux2/2
  Cal2/3(AZ) -> Mux2/3
  Mux2/1 -> [Acceleration]  "acceleration"
  [Acceleration] -> Bus Creator/3
  Mux1/1 -> [Angular_Rate_Uncalibrate]  "omega"
  [Angular_Rate_Uncalibrate] -> Bus Creator/2
  Mux/1 -> [Angle_Uncalibrate]  "angle"
  [Angle_Uncalibrate] -> Bus Creator/1
  Gain1/1 -> Mux1/3
  angle/2 -> Terminator1/1
  angle/4 -> Cal/1(X_L)
  angle/5 -> Cal/2(X_H)
  angle/6 -> Cal/3(Y_L)
  angle/7 -> Cal/4(Y_H)
  angle/8 -> Cal/5(Z_L)
  angle/9 -> Cal/6(Z_H)
  Cal/3(AZ) -> Gain2/1
  omega/2 -> Terminator3/1
  omega/9 -> Cal1/6(Z_H)
  omega/8 -> Cal1/5(Z_L)
  omega/7 -> Cal1/4(Y_H)
  omega/6 -> Cal1/3(Y_L)
  omega/5 -> Cal1/2(X_H)
  omega/4 -> Cal1/1(X_L)
  Cal/2(AY) -> Mux/2
  Cal/1(AX) -> Mux/1
  Cal1/2(AY) -> Mux1/2
  Cal1/1(AX) -> Mux1/1
  omega/3 -> Terminator4/1
  accel/2 -> Terminator7/1
  accel/3 -> Terminator8/1
  accel/4 -> Cal2/1(X_L)
  accel/5 -> Cal2/2(X_H)
  accel/6 -> Cal2/3(Y_L)
  accel/7 -> Cal2/4(Y_H)
  accel/8 -> Cal2/5(Z_L)
  accel/9 -> Cal2/6(Z_H)
  Height/1 -> Cal3/Enable
  Height/2 -> Terminator5/1
  Height/3 -> Terminator6/1
  Height/4 -> Cal3/1(L)
  Height/5 -> Cal3/2(LH)
  Height/6 -> Cal3/3(HL)
  Height/7 -> Cal3/4(H)
  Height/8 -> Terminator9/1
  Height/9 -> Terminator10/1
  Cal3/1(Altitude) -> [Altitude]
  [Altitude] -> Bus Creator/4  "altitude"
  Magnetism/1 -> Cal4/Enable
  Magnetism/2 -> Terminator11/1
  Magnetism/3 -> Terminator12/1
  Magnetism/4 -> Cal4/1(X_L)
  Magnetism/5 -> Cal4/2(X_H)
  Magnetism/6 -> Cal4/3(Y_L)
  Magnetism/7 -> Cal4/4(Y_H)
  Magnetism/8 -> Cal4/5(Z_L)
  Magnetism/9 -> Cal4/6(Z_H)
  Cal4/1(Mag_X) -> Mux3/1
  Cal4/2(Mag_Y) -> Mux3/2
  Cal4/3(Mag_Z) -> Mux3/3
  Mux3/1 -> [Magnetism]  "Magnetism"
  [Magnetism] -> Bus Creator/5
  Bus Creator/1 -> IMU BUS/1
  Gain2/1 -> Mux/3

== system huamo/Orange LED ==
  In1 : Inport
  Blue LED : stm32f4_io_lib/Digital Output  use_bitband=on  port=C  speed=100  porttype=Push Pull  porttypestr=PP  use_pin0=off  use_pin1=off  use_pin2=on  use_pin3=off  use_pin4=off  use_pin5=off  use_pin6=off  use_pin7=off  use_pin8=off  use_pin9=off  use_pin10=off  use_pin11=off  use_pin12=off  use_pin13=off  use_pin14=off  use_pin15=off  pinstr=GPIO_Pin_2  usedpinarray="[0  0  1  0  0  0  0  0  0  0  0  0  0  0  0  0]"  bitbandingstr="#define OrangeLEDBlueLED_C2 Peripheral_BB(GPIOC->ODR, 2)  /* Output pin */"  sampletime=-1  sampletimestr=0.005  blockid=OrangeLEDBlueLED  enablecustomportlabel=off  globalinit=off  cinputportlabel=In1, In2  coutputportlabel=0
  wires:
  In1/1 -> Blue LED/1

== system huamo/Orange LED1 ==
  In1 : Inport
  Blue LED : stm32f4_io_lib/Digital Output  use_bitband=on  port=C  speed=100  porttype=Push Pull  porttypestr=PP  use_pin0=off  use_pin1=off  use_pin2=on  use_pin3=off  use_pin4=off  use_pin5=off  use_pin6=off  use_pin7=off  use_pin8=off  use_pin9=off  use_pin10=off  use_pin11=off  use_pin12=off  use_pin13=off  use_pin14=off  use_pin15=off  pinstr=GPIO_Pin_2  usedpinarray="[0  0  1  0  0  0  0  0  0  0  0  0  0  0  0  0]"  bitbandingstr="#define OrangeLED1BlueLED_C2 Peripheral_BB(GPIOC->ODR, 2)  /* Output pin */"  sampletime=-1  sampletimestr=0.005  blockid=OrangeLED1BlueLED  enablecustomportlabel=off  globalinit=off  cinputportlabel=In1, In2  coutputportlabel=0
  wires:
  In1/1 -> Blue LED/1
